simulink model "rot1"  (R2014b)
settings: Solver=ode15s  StartTime=0.0  StopTime=1.001  RelTol=1e-3
settings Model: Creator=sebastian  LastModifiedBy=li9i

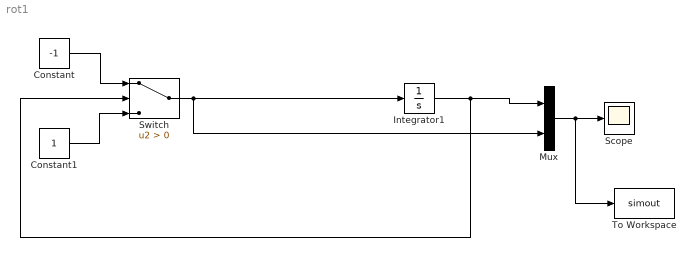
== system rot1 ==
  Constant : Constant  Value=-1
  Constant1 : Constant
  Integrator1 : Integrator  InitialCondition=1
  Mux : Mux  Inputs=2
  Scope : Scope
  Switch : Switch  Criteria=u2 > Threshold  ZeroCross=off
  To Workspace : ToWorkspace  VariableName=simout  SaveFormat=Timeseries  SampleTime=-1
  wires:
  Constant/1 -> Switch/1
  Constant1/1 -> Switch/3
  Mux/1 -> To Workspace/1, Scope/1
  Integrator1/1 -> Mux/1, Switch/2
  Switch/1 -> Integrator1/1, Mux/2
